simulink model "PX10s"  (R2015b)
settings: Solver=VariableStepAuto  StartTime=0.0  StopTime=10.0  RelTol=1e-3
settings Model: Creator=xmax1946  LastModifiedBy=xmax1946

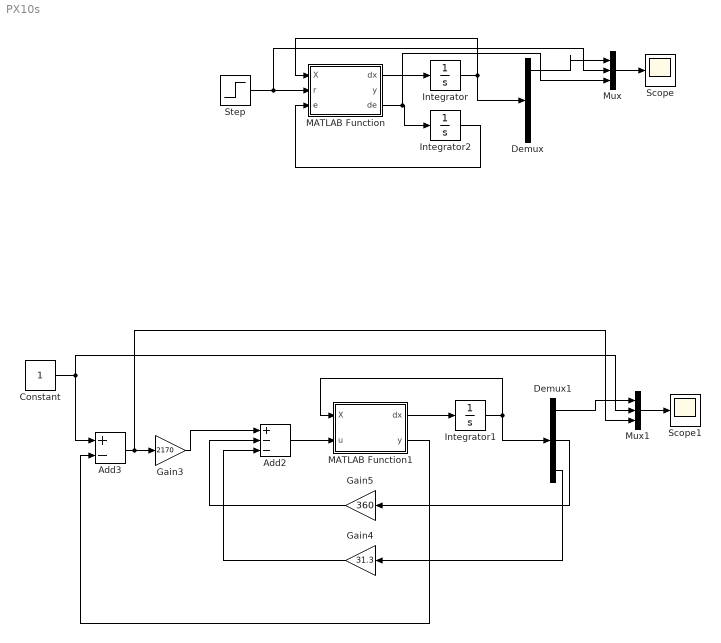
== system PX10s ==
  Add2 : Sum  Inputs=+--
  Add3 : Sum  Inputs=+-
  Constant : Constant
  Demux : Demux  Outputs=3
  Demux1 : Demux  Outputs=3
  Gain3 : Gain  Gain=2170
  Gain4 : Gain  Gain=31.3
  Gain5 : Gain  Gain=360
  Integrator : Integrator  InitialCondition=[0;0;0]
  Integrator1 : Integrator  InitialCondition=[0;0;0]
  Integrator2 : Integrator
  MATLAB Function : MATLAB Function  TreatAsAtomicUnit=on
  MATLAB Function1 : MATLAB Function  TreatAsAtomicUnit=on
  Mux : Mux  Inputs=3
  Mux1 : Mux  Inputs=3
  Scope : Scope
  Scope1 : Scope
  Step : Step  SampleTime=0
  wires:
  MATLAB Function/1(dx) -> Integrator/1
  Integrator/1 -> Demux/1, MATLAB Function/1(X)
  Mux/1 -> Scope/1
  Demux/1 -> Mux/1
  MATLAB Function1/1(dx) -> Integrator1/1
  Integrator1/1 -> Demux1/1, MATLAB Function1/1(X)
  MATLAB Function1/2(y) -> Add3/2
  Demux1/2 -> Gain5/1
  Demux1/3 -> Gain4/1
  Add3/1 -> Mux1/3, Gain3/1
  Add2/1 -> MATLAB Function1/2(u)
  Gain3/1 -> Add2/1
  Gain5/1 -> Add2/2
  Gain4/1 -> Add2/3
  Mux1/1 -> Scope1/1
  Demux1/1 -> Mux1/1
  Constant/1 -> Add3/1, Mux1/2
  MATLAB Function/3(de) -> Mux/3, Integrator2/1
  Integrator2/1 -> MATLAB Function/3(e)
  Step/1 -> Mux/2, MATLAB Function/2(r)

== matlab function PX10s/MATLAB Function1 ==
  data: X input; dx output; u input; y output
function [dx,y] = fcn(X,u)
A=[0,1,0;0,0,1;0,-5,-6];
B=[0;0;1];
C=[1,0,0];

dx=A*X+B*u;
y = C*X;

== matlab function PX10s/MATLAB Function ==
  data: X input; dx output; r input; y output; e input; de output
function [dx,y,de] = fcn(X,r,e)
A=[0,1,0;0,0,1;-1,-5,-6];
B=[0;1;1];
C=[1,0,0];

Ki=285.71;
K=[73.3787,17.6351,.3649];

de=r-C*X;
u=Ki*e-K*X;
dx=A*X+B*u;
y = C*X;
